simulink library "carnot"  (R2018b)
settings: Solver=VariableStepAuto  StartTime=0.0  StopTime=10.0  RelTol=1e-3
undefined symbols (not defined in the file or in its folder): A, A_earth, acol, Acol, ActPower1, ActPower2, ActPower3, Ad, Ad0, Ar, Au, Au0, Azimuth_Angle, B, Bd, Bd0, Br, Bu, Bu0, C, c1, c2, c3, c33, c4, c5, c6, CarnotCallbacks_Density, CarnotCallbacks_Enthalpy, CarnotCallbacks_Enthalpy2Temperature, CarnotCallbacks_Entropy, CarnotCallbacks_Evaporation_Enthalpy, CarnotCallbacks_GlobalMessageLevel, CarnotCallbacks_Grashof, CarnotCallbacks_Heat_Capacity, CarnotCallbacks_Kinematic_Viscosity, CarnotCallbacks_PMV_PPD, CarnotCallbacks_Prandtl, CarnotCallbacks_Saturation_Property, CarnotCallbacks_Saturation_Temperature, CarnotCallbacks_Saturation_Value_Water, CarnotCallbacks_Specific_Volume, CarnotCallbacks_Thermal_Conductivity, CarnotCallbacks_Vapour_Content, CarnotCallbacks_Vapour_Pressure, Cd, Cdl, Cr, Cu, Davies, Dd, DE_TRY2010_04_averageYear, delta_grd, density, DiameterLastPiece, dl, DPConstant, DPLinear, DPQuadratic, Dr ... (+59)
libraries: $bdroot x429, simulink x36, simulink_extras x12
(part 20 of 22)

== system carnot/Source/Chiller/Absorption_Chiller_ddT/boiler ==
  THBhot_in : Inport
  deltadelta_t : Inport  Port=2
  on : Inport  Port=3
  Bus Assignment : BusAssignment  AssignedSignals=Temperature
  Bus Selector : BusSelector  OutputSignals=Temperature,MassFlow,Pressure,FluidType,FluidMix
  Pressure_Drop_Fix : $bdroot/Basic/Pressure_Drop/Pressure_Drop_Fix  con=0  lin=dpg(1)  qua=dpg(2)
  Qdot_G with deltadelta_t : Subsystem
  Thot_out : Subsystem
  prod : Product
  THVhot_out : Outport
  t_B : Outport  Port=2
  Qdot_G [W] : Outport  Port=3
  wires:
  Pressure_Drop_Fix/1 -> THVhot_out/1
  Thot_out/1(Thot_out) -> Bus Assignment/2
  Bus Assignment/1 -> Pressure_Drop_Fix/1
  THBhot_in/1 -> Bus Assignment/1, Bus Selector/1
  Qdot_G with deltadelta_t/1(Qdot_G [W]) -> prod/2
  on/1 -> prod/1
  prod/1 -> Qdot_G [W]/1, Thot_out/3(Qdot_G)
  deltadelta_t/1 -> Qdot_G with deltadelta_t/1(deltadelta_t)
  Bus Selector/5 -> Thot_out/6(mix)  "<FluidMix>"
  Bus Selector/4 -> Thot_out/5(fluid)  "<FluidType>"
  Bus Selector/3 -> Thot_out/4(p)  "<Pressure>"
  Bus Selector/1 -> t_B/1, Thot_out/1(Thot_in)  "<Temperature>"
  Bus Selector/2 -> Thot_out/2(mdot)  "<MassFlow>"

== system carnot/Source/Chiller/Absorption_Chiller_ddT/deltadelta_t ==
  note: deltadelta_t = t_B - (1+E) * t_AC + E * t_E
  t_B : Inport
  t_E : Inport  Port=2
  t_AC : Inport  Port=3
  Add : Sum  Inputs=++-
  Gain : Gain  Gain=1+E
  Gain1 : Gain  Gain=E
  deltadelta_t : Outport
  wires:
  t_AC/1 -> Gain/1
  t_E/1 -> Gain1/1
  Add/1 -> deltadelta_t/1
  t_B/1 -> Add/1
  Gain1/1 -> Add/2
  Gain/1 -> Add/3

== system carnot/Source/Chiller/Absorption_Chiller_ddT/evaporator ==
  THBload_in : Inport
  deltadelta_t : Inport  Port=2
  on : Inport  Port=3
  Bus Assignment : BusAssignment  AssignedSignals=Temperature
  Bus Selector : BusSelector  OutputSignals=Temperature,MassFlow,Pressure,FluidType,FluidMix
  Pressure_Drop_Fix : $bdroot/Basic/Pressure_Drop/Pressure_Drop_Fix  con=0  lin=dpe(1)  qua=dpe(2)
  Qdot_E with deltadelta_t : Subsystem
  Tchilled_out : Subsystem
  prod : Product
  THBload : Outport
  t_E : Outport  Port=2
  Qdot_E [W] : Outport  Port=3
  wires:
  Pressure_Drop_Fix/1 -> THBload/1
  Bus Assignment/1 -> Pressure_Drop_Fix/1
  THBload_in/1 -> Bus Assignment/1, Bus Selector/1
  Qdot_E with deltadelta_t/1(Qdot_E [W]) -> prod/2
  prod/1 -> Qdot_E [W]/1, Tchilled_out/3(Qdot_E)
  on/1 -> prod/1
  Bus Selector/3 -> Tchilled_out/4(p)  "<Pressure>"
  Tchilled_out/1(Tcold) -> Bus Assignment/2, t_E/1
  deltadelta_t/1 -> Qdot_E with deltadelta_t/1(deltadelta_t)
  Bus Selector/5 -> Tchilled_out/6(mix)  "<FluidMix>"
  Bus Selector/4 -> Tchilled_out/5(fluid)  "<FluidType>"
  Bus Selector/1 -> Tchilled_out/1(T)  "<Temperature>"
  Bus Selector/2 -> Tchilled_out/2(mdot)  "<MassFlow>"

== system carnot/Source/Chiller/Compression_Air_Water_Chiller/Lookup_tables _COP + Q_cold_faktor ==
  T_AIR_IN : Inport
  T_WATER_OUT : Inport  Port=2
  control_AC : Inport  Port=3
  Constant : Constant  Value=Q_Nom
  Gain : Gain  Gain=1000
  Product : Product  RndMeth=Zero
  Product1 : Product  Inputs=4  RndMeth=Zero
  Product2 : Product  Inputs=/*  RndMeth=Zero
  lookup_table_COP : Lookup_n-D  BreakpointsForDimension1=[7,18]  BreakpointsForDimension2=[15,20,25,30,35,40]  BreakpointsForDimension3=[1:2]  BreakpointsForDimension4=[1:2]  Table=[3.55 3.15 2.65 2.25 2 1.7;3.8 3.4 2.93 2.58 2.2 1.95]  InputSameDT=on
  lookup_table_Q_cold_faktor : Lookup_n-D  BreakpointsForDimension1=[7,18]  BreakpointsForDimension2=[15,20,25,30,35,40]  BreakpointsForDimension3=[1:2]  BreakpointsForDimension4=[1:2]  Table=|  InputSameDT=on
      | [ 1.26 1.19 1.08 1.00 0.90 0.79;
      |              1.65 1.53 1.41 1.28 1.18 1.09]
  runtime_AC : Subsystem  TreatAsAtomicUnit=on
      mask help: This block counts the time if input is set to one, it stops counting if input is zero and continues when input rises to one again.
      mask Help: eval('filetest (''manual.htm#count_working_time'')')
  start-up-faktor : Fcn  Expr=1-exp(-u/(150/5))
  COP : Outport
  Q_cold : Outport  Port=2
  P_el : Outport  Port=3
  wires:
  Gain/1 -> Q_cold/1, Product2/2
  T_WATER_OUT/1 -> lookup_table_Q_cold_faktor/1, lookup_table_COP/1
  T_AIR_IN/1 -> lookup_table_Q_cold_faktor/2, lookup_table_COP/2
  lookup_table_COP/1 -> Product/1, Product2/1
  control_AC/1 -> Product/2, runtime_AC/1(control_AC), Product1/2
  lookup_table_Q_cold_faktor/1 -> Product1/3
  runtime_AC/1(runtime) -> start-up-faktor/1
  Product/1 -> COP/1
  Product1/1 -> Gain/1
  start-up-faktor/1 -> Product1/1
  Constant/1 -> Product1/4
  Product2/1 -> P_el/1

== system carnot/Source/Chiller/Compression_Air_Water_Chiller/cooling ==
  THB_in : Inport
  Q_cold : Inport  Port=2
  Bus Assignment : BusAssignment  AssignedSignals=Temperature
  Bus Selector : BusSelector  OutputSignals=Temperature,MassFlow
  Constant : Constant  Value=20
  Constant_THB : $bdroot/Source/Simple/Constant_THB  t=40  mdot=0*100/3600  p=1e5  mID=No Pressure Drop  fluid=Water  mix=0  mix2=0  mix3=0  dia=0.02  hgt=0
  Ground : Ground
  Heat_Capacity : $bdroot/Basic/Material_Properties/Heat_Capacity  VariantControl=CarlibClassic  INPUTARGUMENTS=THB  DEBUGLEVEL=DEBUGLEVEL  MAXTOTALWARNINGS=inf  MAXCONSECUTIVEWARNINGS=inf  WRITETOFILE=0  FILENAME='errors.txt'
  Product : Product  Inputs=//*  SaturateOnIntegerOverflow=on  RndMeth=Zero  InputSameDT=on  OutDataTypeStr=Inherit: Same as first input
  Saturation : Saturate  UpperLimit=inf  LowerLimit=1
  Storage_Type_1 : $bdroot/Storage/Thermal/Storage_Type_1  t0=20  hgt=1.7684  stgtype=1  tini=[20 20 20 20 20 20 20 20 20 20]  mpts=[1 2 3 4 5 6 7 8 9 10]  PathName=fullfile(path_carnot('libsl'), 'Storage', 'Thermal', 'Storage_Type_1', 'parameter_set')  FileName='StorageType1_500_L.mat'  userPath=off  userParam=off  uwall=1  ubot=1  utop=1  axcond=1  volume=0.5  dia=0.6  standing=standing cylinder  nodes=10  mpoints=10  Tsensor=0.5  pipe1inlet=1  pipe1outlet=0  pipe1dia=0.03  pipe2inlet=0  pipe2outlet=1  pipe2dia=0.03  heater1start=0.6  heater1end=0.65
  Sum2 : Sum  Inputs=+-  InputSameDT=on  OutDataTypeStr=Inherit: Same as first input
  Terminator : Terminator
  Terminator1 : Terminator
  Terminator2 : Terminator
  isinf : MATLAB Function  TreatAsAtomicUnit=on
  isnan : MATLAB Function  TreatAsAtomicUnit=on
  THB_out : Outport
  wires:
  Ground/1 -> Storage_Type_1/4
  Storage_Type_1/3 -> Terminator2/1
  Storage_Type_1/2 -> Terminator1/1
  Storage_Type_1/1 -> Terminator/1
  Storage_Type_1/4 -> THB_out/1
  Bus Selector/2 -> Product/1  "<MassFlow>"
  Heat_Capacity/1 -> Product/2
  Bus Assignment/1 -> Storage_Type_1/3
  Constant/1 -> Storage_Type_1/1
  Constant_THB/1 -> Storage_Type_1/2
  THB_in/1 -> Heat_Capacity/1, Bus Selector/1, Bus Assignment/1
  Bus Selector/1 -> Sum2/1  "<Temperature>"
  Q_cold/1 -> Product/3  "W"
  isnan/1(y) -> isinf/1(u)
  Product/1 -> isnan/1(u)
  isinf/1(y) -> Sum2/2
  Sum2/1 -> Saturation/1
  Saturation/1 -> Bus Assignment/2

== system carnot/Source/Chiller/Compression_Air_Water_Chiller/measure_T_WATER_OUT ==
  THV_in : Inport
  Demux3 : Demux  Outputs=2
  Terminator : Terminator
  heat capacity : StateSpace  A=-tc  B=tc  D=0  InitialCondition=t0
  select temperature : Selector  InputPortWidth=5  IndexOptions=Index vector (dialog)  Indices=[2]  OutputSizes=1
  T : Outport
  THV : Outport  Port=2
  wires:
  Demux3/2 -> Terminator/1
  Demux3/1 -> select temperature/1
  THV_in/1 -> Demux3/1, THV/1
  select temperature/1 -> heat capacity/1
  heat capacity/1 -> T/1

== system carnot/Source/Chiller/Cooling_Tower/Fan ==
  note: Grundlage zur Berechnung
      | bei Drehzahländerung eines bestimmten Lüfters
      |
      | Proportionalitätsgesetz
      | V1/V2 = n1/n2
      | P1/P2 = (n1/n2)^3
      |
      | Wirkungsgrad Elektromotor
      | P = Pm/eta
  n_fan : Inport
  Divide1 : Product  Inputs=*/
  Divide2 : Product  Inputs=*/*
  Divide3 : Product  Inputs=/*
  Divide4 : Product  Inputs=/*
  Input Leistung : Constant  Value=1.8
  Math Function : Math  Operator=pow  SaturateOnIntegerOverflow=on
  Pw1 : Constant  Value=3
  max. Drehzahl : Constant  Value=824
  max. Vdot_Lüfter : Constant  Value=2.2
  n_fan [%] : Outport
  vdot_fan : Outport  Port=2
  P_fan : Outport  Port=3
  wires:
  n_fan/1 -> Divide2/1, Divide4/1, Divide1/1
  max. Drehzahl/1 -> Divide2/2, Divide1/2, Divide4/2
  Divide1/1 -> n_fan [%]/1
  Input Leistung/1 -> Divide3/2
  max. Vdot_Lüfter/1 -> Divide2/3
  Divide2/1 -> vdot_fan/1
  Divide3/1 -> P_fan/1
  Divide4/1 -> Math Function/1
  Math Function/1 -> Divide3/1
  Pw1/1 -> Math Function/2

== system carnot/Source/Chiller/Cooling_Tower/Feuchtkugel- temperatureinfluss // wet-bulb temperature effect ==
  WDB : Inport
  t_ie : Inport  Port=2
  Enable : EnablePort
  "Abgleich " : Subsystem
  Add : Sum
  Constant : Constant  Value=2
  Divide : Product  Inputs=*/
  THB_WetBulbTemperature : $bdroot/Basic/Material_Properties/THB_WetBulbTemperature
  Terminator1 : Terminator
  WDB2THB : $bdroot/Weather/WDB2THB  dia=0.2
  wet-bulb 15 °C : Subsystem
  t_FK : Outport  InitialOutput=0
  t_ia_FK : Outport  Port=2  InitialOutput=0
  dt : Outport  Port=3  InitialOutput=0
  wires:
  WDB2THB/1 -> THB_WetBulbTemperature/1
  THB_WetBulbTemperature/2 -> Terminator1/1
  WDB/1 -> WDB2THB/1
  wet-bulb 15 °C/1(t_ia_FK15) -> "Abgleich "/3(t_ia_FK15)
  THB_WetBulbTemperature/1 -> "Abgleich "/1(t_FK), t_FK/1
  t_ie/1 -> Add/2, wet-bulb 15 °C/1(t_ie), "Abgleich "/2(t_ie)
  "Abgleich "/1(t_ia_FK) -> Add/1, t_ia_FK/1
  Add/1 -> Divide/1
  Constant/1 -> Divide/2
  Divide/1 -> dt/1

== system carnot/Source/Chiller/Cooling_Tower/Leistungseinflüsse // influence on coolingpower ==
  t_ia_FK : Inport
  cp_i : Inport  Port=2
  t_ie : Inport  Port=3
  mdot_i : Inport  Port=4
  Fluid_Type : Inport  Port=5
  Fluid_mix : Inport  Port=6
  n_fan [%] : Inport  Port=7
  Enable : EnablePort
  Qdot_i_FK : Subsystem
  "Qdot_i_ist " : Subsystem
  "t_ia_ist " : Subsystem
  Qdot_i_ist : Outport  InitialOutput=0
  t_ia_ist : Outport  Port=2  InitialOutput=0
  wires:
  "Qdot_i_ist "/1(Qdot_i_ist) -> Qdot_i_ist/1, "t_ia_ist "/1(Qdot_i_ist)
  Qdot_i_FK/1(Qdot_i_FK) -> "Qdot_i_ist "/1(Qdot_i_FK)
  t_ie/1 -> Qdot_i_FK/2(t_ie), "t_ia_ist "/2(t_ie), "Qdot_i_ist "/6(t_ie)
  t_ia_FK/1 -> Qdot_i_FK/1(t_ia_FK)
  n_fan [%]/1 -> "Qdot_i_ist "/2(n_Fan [%])
  "t_ia_ist "/1(t_ia_ist) -> t_ia_ist/1
  cp_i/1 -> "t_ia_ist "/3(cp_i)
  Fluid_Type/1 -> Qdot_i_FK/3(Fluid_Type), "Qdot_i_ist "/5(Fluid_Type)
  mdot_i/1 -> "Qdot_i_ist "/4(mdot_i), "t_ia_ist "/4(mdot)
  Fluid_mix/1 -> "Qdot_i_ist "/3(Fluid_mix)

== system carnot/Source/Chiller/Cooling_Tower/Verbrauch // consumption ==
  Qdot : Inport
  vdot_fan : Inport  Port=2
  P_fan : Inport  Port=3
  control_fan : Inport  Port=4
  phi_le : Inport  Port=5
  t_le : Inport  Port=6
  t_ie : Inport  Port=7
  Strom : Subsystem
  Verdunstung : Subsystem
  energy : Outport
  power : Outport  Port=2
  Wasserverbrauch : Outport  Port=3
  wires:
  control_fan/1 -> Strom/1(control_Fan), Verdunstung/1(control_Fan)
  P_fan/1 -> Strom/2(P_Fan)
  Strom/2(power) -> power/1
  t_le/1 -> Verdunstung/2(t_le)
  Verdunstung/1(Wasserverbrauch) -> Wasserverbrauch/1
  phi_le/1 -> Verdunstung/3(phi_le)
  vdot_fan/1 -> Verdunstung/4(Vdot_Fan)
  Qdot/1 -> Verdunstung/5(Qdot)
  t_ie/1 -> Verdunstung/6(t_ie)
  Strom/1(energy) -> energy/1

== system carnot/Source/Cogeneration/microCHP_constant/energy and efficiency ==
  P_th : Inport
  control_CHP : Inport  Port=2
  P_gas : Inport  Port=3
  P_el : Inport  Port=4
  Add : Sum
  Dot Product1 : DotProduct  InputSameDT=on  OutDataTypeStr=Inherit: Inherit via internal rule
  Dot Product2 : DotProduct  InputSameDT=on  OutDataTypeStr=Inherit: Inherit via internal rule
  Dot Product4 : DotProduct  InputSameDT=on  OutDataTypeStr=Inherit: Inherit via internal rule
  Integrator : Integrator
  Integrator1 : Integrator
  Integrator2 : Integrator
  Product1 : Product  Inputs=*/  SaturateOnIntegerOverflow=on  RndMeth=Zero  InputSameDT=on  OutDataTypeStr=Inherit: Same as first input
  Product2 : Product  Inputs=/*  SaturateOnIntegerOverflow=on  RndMeth=Zero  InputSameDT=on  OutDataTypeStr=Inherit: Same as first input
  Q_th : Outport
  Q_el : Outport  Port=2
  Q_Gas : Outport  Port=3
  eta_th : Outport  Port=4
  eta_el : Outport  Port=5
  eta_sys : Outport  Port=6
  wires:
  Add/1 -> eta_sys/1
  Product1/1 -> eta_th/1, Add/1
  Integrator1/1 -> Q_th/1, Product1/1
  P_th/1 -> Dot Product1/1
  Dot Product1/1 -> Integrator1/1
  Integrator2/1 -> Q_el/1, Product2/2
  Integrator/1 -> Product1/2, Q_Gas/1, Product2/1
  control_CHP/1 -> Dot Product1/2, Dot Product4/1, Dot Product2/1
  Dot Product2/1 -> Integrator/1
  Dot Product4/1 -> Integrator2/1
  Product2/1 -> Add/2, eta_el/1
  P_el/1 -> Dot Product4/2
  P_gas/1 -> Dot Product2/2

== system carnot/Source/Cogeneration/microCHP_constant/measure_T ==
  THV_in : Inport
  heat capacity : StateSpace  A=-tc  B=tc  D=0  InitialCondition=t0
  select temperature : Selector  InputPortWidth=20  IndexOptions=Index vector (dialog)  Indices=[2]  OutputSizes=1
  THV : Outport
  T : Outport  Port=2
  wires:
  heat capacity/1 -> T/1
  select temperature/1 -> heat capacity/1
  THV_in/1 -> THV/1, select temperature/1

== system carnot/Source/Cogeneration/microCHP_constant/pump and return temperature raising facility ==
  note: heating power
  THVin : Inport
  control : Inport  Port=2
  " " : Constant  Value=P_th
  " ." : Product  Inputs=*/
  " .  " : Sum  Inputs=-+
  . : Sum  Inputs=-+
  ". " : Product  Inputs=*/
  Demux : Demux  Outputs=[1 1 18]
  Divide1 : Product  Inputs=****
  Ground : Ground
  Mux1 : Mux  Inputs=[1 1 1 7 10]
  P_th_base : Constant  Value=11520
  T_flow-lookup table : Lookup_n-D  NumberOfTableDimensions=1  BreakpointsForDimension1=[45,50,60,65,74]  BreakpointsForDimension2=[44,80]  BreakpointsForDimension3=[1:2]  BreakpointsForDimension4=[1:2]  Table=[78.5 79.65 81 84.18 92.47]  InputSameDT=on
  T_flow_setpoint : Constant  Value=T_flow_setpoint
  const1 : Constant  Value=[p0 fluid_id mix dia 0 0 0]
  heat capacity : Subsystem  mask{NTU=3.3}
      mask prompts: NTU "NTU (k*A/(m*cp))"
  mass flow-lookup table : Lookup_n-D  NumberOfTableDimensions=1  BreakpointsForDimension1=[45,50,60,65,74]  BreakpointsForDimension2=[44,80]  BreakpointsForDimension3=[1:2]  BreakpointsForDimension4=[1:2]  Table=[0.09 0.1 0.129 0.139 0.140]  InputSameDT=on
  terminate1 : Terminator
  THV : Outport
  wires:
  control/1 -> Divide1/4
  " ."/1 -> Divide1/3  "f_power"
  ". "/1 -> Divide1/2  "f_flowSetpoint"
  P_th_base/1 -> " ."/2
  T_flow-lookup table/1 -> ./2
  T_flow_setpoint/1 -> " .  "/2
  " .  "/1 -> ". "/2
  ./1 -> ". "/1
  Divide1/1 -> Mux1/3  "mdot"
  mass flow-lookup table/1 -> Divide1/1
  " "/1 -> " ."/1
  THVin/1 -> Demux/1
  const1/1 -> Mux1/4
  Demux/3 -> terminate1/1
  heat capacity/1(T) -> Mux1/2
  Demux/2 -> " .  "/1, T_flow-lookup table/1, ./1, mass flow-lookup table/1, heat capacity/1(Tin)  "T"
  Mux1/1 -> THV/1
  Demux/1 -> Mux1/1  "ID"
  Ground/1 -> Mux1/5  "not used"

== system carnot/Source/Cogeneration/microCHP_modulating/Control_Unit ==
  note: T_flow_ctrl
  cp : Inport
  mdot_return : Inport  Port=2
  T_flow : Inport  Port=3
  demand_control : Inport  Port=4
  T_return_load : Inport  Port=5
  Add : Sum  Inputs=+-
  Constant1 : Constant  Value=60
  Constant10 : Constant  Value=T_flow_setpoint
  Constant6 : Constant
  Constant7 : Constant  Value=t_start
  Constant8 : Constant  Value=P_th_start
  Constant9 : Constant  Value=P_th_max
  Integrator : Integrator  ExternalReset=level
  Logical Operator1 : Logic  Operator=NOT  AllPortsSameDT=off  OutDataTypeStr=boolean
  MinMax : MinMax  Inputs=2
  Product : Product
  Product1 : Product  Inputs=3
  Relational Operator : RelationalOperator  Operator=>  OutDataTypeStr=boolean  RndMeth=Simplest
  Relational Operator1 : RelationalOperator  Operator=>  OutDataTypeStr=boolean  RndMeth=Simplest
  Relay : Relay  OnSwitchValue=T_flow_max  OffSwitchValue=T_flow_max-1  OnOutputValue=0  OffOutputValue=1
  Saturation : Saturate  UpperLimit=P_th_max  LowerLimit=P_th_min
  Switch1 : Switch  Criteria=u2 ~= 0
  Switch2 : Switch  Criteria=u2 ~= 0
  control_CHP : Outport
  P_th : Outport  Port=2
  wires:
  T_return_load/1 -> Add/2
  cp/1 -> Product1/2
  Product/1 -> P_th/1
  mdot_return/1 -> Product1/1
  demand_control/1 -> MinMax/2
  T_flow/1 -> Relay/1, Relational Operator/1
  Add/1 -> Product1/3
  Relay/1 -> MinMax/1
  MinMax/1 -> control_CHP/1, Product/2, Logical Operator1/1
  Constant1/1 -> Relational Operator/2
  Relational Operator/1 -> Switch1/2
  Saturation/1 -> Switch1/1  "Pth_setpoint"
  Constant6/1 -> Integrator/1
  Logical Operator1/1 -> Integrator/2
  Integrator/1 -> Relational Operator1/1
  Constant7/1 -> Relational Operator1/2
  Relational Operator1/1 -> Switch2/2
  Constant8/1 -> Switch2/3
  Constant9/1 -> Switch1/3
  Switch1/1 -> Switch2/1
  Constant10/1 -> Add/1
  Product1/1 -> Saturation/1
  Switch2/1 -> Product/1

== system carnot/Source/Cogeneration/microCHP_modulating/energy and efficiency ==
  control CHP : Inport
  P_th : Inport  Port=2
  P_gas : Inport  Port=3
  P_el : Inport  Port=4
  Add : Sum
  Dot Product1 : DotProduct  InputSameDT=on  OutDataTypeStr=Inherit: Inherit via internal rule
  Dot Product2 : DotProduct  InputSameDT=on  OutDataTypeStr=Inherit: Inherit via internal rule
  Dot Product4 : DotProduct  InputSameDT=on  OutDataTypeStr=Inherit: Inherit via internal rule
  Integrator : Integrator
  Integrator1 : Integrator
  Integrator2 : Integrator
  Product1 : Product  Inputs=*/  SaturateOnIntegerOverflow=on  RndMeth=Zero  InputSameDT=on  OutDataTypeStr=Inherit: Same as first input
  Product2 : Product  Inputs=/*  SaturateOnIntegerOverflow=on  RndMeth=Zero  InputSameDT=on  OutDataTypeStr=Inherit: Same as first input
  Q_th : Outport
  Q_el : Outport  Port=2
  Q_gas : Outport  Port=3
  eta_th : Outport  Port=4
  eta_el : Outport  Port=5
  eta_sys : Outport  Port=6
  wires:
  P_gas/1 -> Dot Product2/2
  P_el/1 -> Dot Product4/2
  Product2/1 -> eta_el/1, Add/2
  Dot Product4/1 -> Integrator2/1
  Dot Product2/1 -> Integrator/1
  control CHP/1 -> Dot Product2/1, Dot Product4/1, Dot Product1/2
  Integrator/1 -> Product2/1, Q_gas/1, Product1/2
  Integrator2/1 -> Product2/2, Q_el/1
  Dot Product1/1 -> Integrator1/1
  P_th/1 -> Dot Product1/1
  Integrator1/1 -> Product1/1, Q_th/1
  Product1/1 -> Add/1, eta_th/1
  Add/1 -> eta_sys/1

== system carnot/Source/Cogeneration/microCHP_modulating/measure_T ==
  THV_in : Inport
  heat capacity : StateSpace  A=-tc  B=tc  D=0  InitialCondition=t0
  select temperature : Selector  InputPortWidth=20  IndexOptions=Index vector (dialog)  Indices=[2]  OutputSizes=1
  T : Outport
  THV : Outport  Port=2
  wires:
  THV_in/1 -> select temperature/1, THV/1
  select temperature/1 -> heat capacity/1
  heat capacity/1 -> T/1

== system carnot/Source/Cogeneration/microCHP_modulating/measure_mdot ==
  THV_in : Inport
  select massflow : Selector  InputPortWidth=20  IndexOptions=Index vector (dialog)  Indices=[3]  OutputSizes=1
  THV : Outport
  mdot : Outport  Port=2
  wires:
  THV_in/1 -> select massflow/1, THV/1
  select massflow/1 -> mdot/1

== system carnot/Source/Cogeneration/microCHP_modulating/pump_const ==
  note: maximum power
  note: nominal power of basic unit
  THVin : Inport
  control : Inport  Port=2
  Constant : Constant  Value=P_th_max
  Constant2 : Constant  Value=12500
  Demux1 : Demux  Outputs=[1 1 18]
  Ground : Ground
  ID : Constant
  Mux1 : Mux  Inputs=[1 1 1 7 10]
  Product1 : Product  Inputs=**/  SaturateOnIntegerOverflow=on  RndMeth=Zero  InputSameDT=on  OutDataTypeStr=Inherit: Same as first input
  Terminator : Terminator
  const1 : Constant  Value=[p0 fluid_id mix dia 0 0 0]
  heat capacity : Subsystem  mask{NTU=3.1}
      mask prompts: NTU "NTU (k*A/(m*cp))"
  mdot : Gain  Gain=mdotmax  SaturateOnIntegerOverflow=on  OutDataTypeStr=Inherit: Same as input  ParamDataTypeStr=Inherit: Same as input
  terminate : Terminator
  THV : Outport
  wires:
  Ground/1 -> Mux1/5  "not used"
  Demux1/3 -> terminate/1
  THVin/1 -> Demux1/1
  ID/1 -> Mux1/1  "ID"
  Mux1/1 -> THV/1
  const1/1 -> Mux1/4
  Demux1/1 -> Terminator/1  "ID"
  Demux1/2 -> heat capacity/1(Tin)  "T"
  mdot/1 -> Product1/2
  Constant/1 -> Product1/1
  Constant2/1 -> Product1/3
  Product1/1 -> Mux1/3
  heat capacity/1(T) -> Mux1/2  "T"
  control/1 -> mdot/1

== system carnot/Source/Cogeneration/microCHP_modulating/return temperature raising facility ==
  THB_flow : Inport
  P_th : Inport  Port=2
  THB_return_load : Inport  Port=3
  . : Product  Inputs=//*  SaturateOnIntegerOverflow=on  RndMeth=Zero  InputSameDT=on  OutDataTypeStr=Inherit: Same as first input
  Add : Sum  Inputs=+-
  Bus Selector : BusSelector  OutputSignals=MassFlow,Temperature,Pressure,FluidType,FluidMix
  Constant1 : Constant  Value=T_flow_setpoint
  Constant3 : Constant  Value=0
  Flow_Diverter : $bdroot/Hydraulics/Flow_Diverter
  Flow_Mixer_Thermostatic : $bdroot/Hydraulics/Flow_Mixer_Thermostatic  t=1
  Heat_Capacity : $bdroot/Basic/Material_Properties/Heat_Capacity  VariantControl=CarlibClassic  INPUTARGUMENTS=state variables (classic)  DEBUGLEVEL=DEBUGLEVEL  MAXTOTALWARNINGS=inf  MAXCONSECUTIVEWARNINGS=inf  WRITETOFILE=0  FILENAME='errors.txt'
  Switch : Switch  Threshold=1  SaturateOnIntegerOverflow=on  InputSameDT=on
  THB_return : Outport
  THB_flow_load : Outport  Port=2
  wires:
  P_th/1 -> ./3, Switch/2
  Heat_Capacity/1 -> ./2
  Bus Selector/2 -> Heat_Capacity/1  "<Temperature>"
  Bus Selector/1 -> ./1  "<MassFlow>"
  Bus Selector/5 -> Heat_Capacity/4  "<FluidMix>"
  Bus Selector/4 -> Heat_Capacity/3  "<FluidType>"
  Bus Selector/3 -> Heat_Capacity/2  "<Pressure>"
  Flow_Diverter/2 -> THB_flow_load/1
  THB_return_load/1 -> Flow_Mixer_Thermostatic/2
  Constant1/1 -> Add/1
  Add/1 -> Switch/1
  ./1 -> Add/2
  Constant3/1 -> Switch/3
  Switch/1 -> Flow_Mixer_Thermostatic/4
  THB_flow/1 -> Flow_Diverter/1, Bus Selector/1
  Flow_Mixer_Thermostatic/2 -> Flow_Diverter/2
  Flow_Mixer_Thermostatic/1 -> THB_return/1
  Flow_Diverter/1 -> Flow_Mixer_Thermostatic/1
  Flow_Diverter/3 -> Flow_Mixer_Thermostatic/3

== system carnot/Source/Cogeneration/microCHP_modulating/scale_function ==
  P_th : Inport
  . : Sum  Inputs=+-
  .1 : Sum  Inputs=-+
  Add : Sum
  Divide : Product  Inputs=*/
  b : Constant  Value=P_th_max
  m : Constant  Value=P_th_min
  m2 : Constant
  X_pth : Outport
  wires:
  m2/1 -> Add/2
  m/1 -> ./2, .1/1
  ./1 -> Divide/1
  b/1 -> .1/2
  .1/1 -> Divide/2
  P_th/1 -> ./1
  Divide/1 -> Add/1
  Add/1 -> X_pth/1

== system carnot/Source/Heat_Exchanger/Radiator_AIV/Troom ==
  "[AIV]" : Inport
  Sum4 : Sum  Inputs=1  SaturateOnIntegerOverflow=on  InputSameDT=on  OutDataTypeStr=Inherit: Same as first input
  gain : Gain  Gain=0.5  SaturateOnIntegerOverflow=on  OutDataTypeStr=Inherit: Same as input  ParamDataTypeStr=Inherit: Same as input
  select Tc Tr : Selector  InputPortWidth=9  IndexOptions=Index vector (dialog)  Indices=[2 3]  OutputSizes=1
  Troom : Outport
  wires:
  select Tc Tr/1 -> Sum4/1
  Sum4/1 -> gain/1
  gain/1 -> Troom/1  "Troom"
  "[AIV]"/1 -> select Tc Tr/1

== system carnot/Source/Heat_Pump/Ground_Source_Heat_Exchanger/BoundaryCondition1 ==
  note: virtual fluid temperature node T_Earth(i,0) is the
      | fluid temperature that would pull the thermal
      | power through the resistance L1 (= average of
      | Tup and Tdown)
  T_Up : Inport
  T_Down : Inport  Port=2
  T_Earth(i,1) : Inport  Port=3
  Gain : Gain  Gain=1/dl
  Gain1 : Gain  Gain=L1/2  SaturateOnIntegerOverflow=on  OutDataTypeStr=Inherit: Same as input  ParamDataTypeStr=Inherit: Same as input
  Gain2 : Gain  Gain=L1/2  SaturateOnIntegerOverflow=on  OutDataTypeStr=Inherit: Same as input  ParamDataTypeStr=Inherit: Same as input
  Gain3 : Gain  Gain=1/L1  SaturateOnIntegerOverflow=on  OutDataTypeStr=Inherit: Same as input  ParamDataTypeStr=Inherit: Same as input
  Sum3 : Sum  Inputs=|-+  SaturateOnIntegerOverflow=on  InputSameDT=on  OutDataTypeStr=Inherit: Same as first input
  Sum4 : Sum  Inputs=|-+  SaturateOnIntegerOverflow=on  InputSameDT=on  OutDataTypeStr=Inherit: Same as first input
  Sum5 : Sum  Inputs=|++  SaturateOnIntegerOverflow=on  InputSameDT=on  OutDataTypeStr=Inherit: Same as first input
  Sum6 : Sum  Inputs=|-+  SaturateOnIntegerOverflow=on  InputSameDT=on  OutDataTypeStr=Inherit: Same as first input
  T_Earth(i,0) : Outport
  qdot,i : Outport  Port=2
  wires:
  Gain/1 -> qdot,i/1
  Sum6/1 -> T_Earth(i,0)/1
  T_Earth(i,1)/1 -> Sum4/2, Sum6/2, Sum3/2
  T_Up/1 -> Sum4/1
  T_Down/1 -> Sum3/1
  Gain3/1 -> Sum6/1  "dT"
  Sum5/1 -> Gain3/1, Gain/1  "Qtot,i"
  Gain2/1 -> Sum5/2  "Qup,i"
  Gain1/1 -> Sum5/1  "Qdown,i"
  Sum4/1 -> Gain2/1
  Sum3/1 -> Gain1/1

== system carnot/Source/Heat_Pump/Ground_Source_Heat_Exchanger/BoundaryCondition2 ==
  note: T_Earth(i,DimRad)
  qdot,i : Inport
  Dd6 : Gain  Gain=c4  Multiplication=Matrix(K*u)  SaturateOnIntegerOverflow=on  OutDataTypeStr=Inherit: Same as input  ParamDataTypeStr=Inherit: Same as input
  Sum2 : Sum  Inputs=|+-  SaturateOnIntegerOverflow=on  InputSameDT=on  OutDataTypeStr=Inherit: Same as first input
  Tearth DimRad : Constant  Value=T_null  VectorParams1D=off
  g-function : Subsystem
  T_Earth(i,DimRad) Gew : Outport
  T_Earth(i,DimRad) : Outport  Port=2
  wires:
  Sum2/1 -> Dd6/1, T_Earth(i,DimRad)/1
  Tearth DimRad/1 -> Sum2/1
  qdot,i/1 -> g-function/1(qdot,i)
  Dd6/1 -> T_Earth(i,DimRad) Gew/1
  g-function/1(DeltaT) -> Sum2/2  "DeltaT"

== system carnot/Source/Heat_Pump/Ground_Source_Heat_Exchanger/Tdown ==
  note: instationary calculation of Tdown (Huber 1997)
  Tin,TEarth : Inport
  A mult : Product  Multiplication=Matrix(*)  RndMeth=Zero
  B mult : Product  Multiplication=Matrix(*)  RndMeth=Zero
  C mult : Product  Multiplication=Matrix(*)  RndMeth=Zero
  D mult : Product  Multiplication=Matrix(*)  RndMeth=Zero
  Integrator : Integrator  InitialCondition=Tdown_0
  Sum1 : Sum  Inputs=|++
  Sum2 : Sum  Inputs=++|
  Tdown : Outport
  wires:
  Sum2/1 -> Tdown/1  "y"
  Tin,TEarth/1 -> B mult/2, D mult/2
  D mult/1 -> Sum2/1
  C mult/1 -> Sum2/2
  B mult/1 -> Sum1/1
  Sum1/1 -> Integrator/1  "Xdot"
  Integrator/1 -> A mult/2, C mult/2  "X"
  A mult/1 -> Sum1/2
  [B] -> B mult/1
  [A] -> A mult/1
  [C] -> C mult/1
  [D] -> D mult/1

== system carnot/Source/Heat_Pump/Ground_Source_Heat_Exchanger/Tup ==
  note: instationary calculation of Tup (Huber 1997)
  Tin,TEarth : Inport
  A mult : Product  Multiplication=Matrix(*)  RndMeth=Zero
  B mult : Product  Multiplication=Matrix(*)  RndMeth=Zero
  C mult : Product  Multiplication=Matrix(*)  RndMeth=Zero
  D mult : Product  Multiplication=Matrix(*)  RndMeth=Zero
  Integrator : Integrator  InitialCondition=Tup_0
  Sum1 : Sum  Inputs=|++
  Sum2 : Sum  Inputs=++|
  Tup : Outport
  wires:
  Sum2/1 -> Tup/1  "y"
  Tin,TEarth/1 -> B mult/2, D mult/2
  D mult/1 -> Sum2/1
  C mult/1 -> Sum2/2
  B mult/1 -> Sum1/1
  Sum1/1 -> Integrator/1  "Xdot"
  Integrator/1 -> A mult/2, C mult/2  "X"
  A mult/1 -> Sum1/2
  [Bu] -> B mult/1
  [Au] -> A mult/1
  [Cu] -> C mult/1
  [Du] -> D mult/1

== system carnot/Source/Solar_Thermal/Collector_1xN/create_Cdat ==
  acol : Inport
  THBin : Inport  Port=2
  THBout : Inport  Port=3
  Qdot : Inport  Port=4
  Tmean : Inport  Port=5
  WDB : Inport  Port=6
  Bus Creator : BusCreator  Inputs=6
  data_c : Outport
  wires:
  Tmean/1 -> Bus Creator/5  "Tmean"
  Qdot/1 -> Bus Creator/4  "Qdot"
  Bus Creator/1 -> data_c/1
  WDB/1 -> Bus Creator/6  "WDB_surface"
  THBout/1 -> Bus Creator/3  "THBout"
  THBin/1 -> Bus Creator/2  "THBin"
  acol/1 -> Bus Creator/1  "Acol"

== system carnot/Source/Solar_Thermal/Collector_Unglazed/Collector_Unglazed ==
  WDB : Inport
  position : Inport  Port=2
  THB_r : Inport  Port=3
  Add : Sum  Inputs=1
  Bus Assignment : BusAssignment  AssignedSignals=Temperature
  Bus Selector : BusSelector  OutputSignals=Solar_Radiation_direct_surface,Solar_Radiation_diffuse_surface,Temperature_Ambient,Temperature_Sky_Radiation,Relative_Humidity,Station_Pressure,Wind_Speed  OutputAsBus=on
  Bus Selector1 : BusSelector  OutputSignals=Temperature,MassFlow,Pressure,FluidType,FluidMix  OutputAsBus=on
  IAM_Table : $bdroot/Source/Solar_Thermal/IncidenceAngleModifier/IAM_Table  fta=fta  angle=[0:5:90]  Kb="[1.0000    1.0000    0.9999    0.9996    0.9991    0.9982    0.9965  0.9935    0.9886    0.9807    0.9678    0.9473    0.9148    0.8638   0.7846    0.6644    0.4907    0.2599    0.0000]"  Kd=0.92
  PowerMeter : $bdroot/Control/PowerMeter
  Pressure_Drop_Collector : $bdroot/Basic/Pressure_Drop/Pressure_Drop_Collector  len=len  lin=lin  qua=qua
  Product : Product  Inputs=*/  RndMeth=Zero
  Radiation_on_Inclined_Surface : $bdroot/Weather/Radiation_on_Inclined_Surface  sky=Perez 1990  reflect=0.2
  Terminator : Terminator
  Width : Width
  const : Constant  Value=acol
  create_Cdat : Subsystem
  unglazed_collector : S-Function  FunctionName=solarcollector_unglazed  Parameters=acol, uc0, uc1, uc0loss, uc1loss, uc0gain, uc1gain, e_sky, uc1eta0, hi, inv_c_abs, inv_c_fl, len, tini, nodes  SFunctionDeploymentMode=off  EnableBusSupport=off
  Cdat : Outport
  THB_s : Outport  Port=2
  wires:
  IAM_Table/1 -> unglazed_collector/2
  Bus Assignment/1 -> Pressure_Drop_Collector/2, PowerMeter/1
  Radiation_on_Inclined_Surface/1 -> create_Cdat/6(WDB), Bus Selector/1, IAM_Table/1
  position/1 -> Pressure_Drop_Collector/3, Radiation_on_Inclined_Surface/2
  WDB/1 -> Radiation_on_Inclined_Surface/1
  THB_r/1 -> Bus Selector1/1, Bus Assignment/1, create_Cdat/2(THBin), PowerMeter/2
  Bus Selector/1 -> unglazed_collector/1
  Bus Selector1/1 -> unglazed_collector/3
  IAM_Table/2 -> Terminator/1
  unglazed_collector/1 -> Bus Assignment/2
  unglazed_collector/2 -> Add/1, Width/1  "Tabsorber"
  const/1 -> create_Cdat/1(acol)
  create_Cdat/1(data_c) -> Cdat/1  "Cdat"
  PowerMeter/1 -> create_Cdat/4(Qdot)
  Add/1 -> Product/1
  Product/1 -> create_Cdat/5(Tmean)
  Width/1 -> Product/2
  Pressure_Drop_Collector/1 -> create_Cdat/3(THBout), THB_s/1  "THB_s"
  unglazed_collector/3 -> Pressure_Drop_Collector/1  "Tfluid"

== system carnot/Source/Solar_Thermal/Collector_Unglazed_ISO9806/create_Cdat ==
  acol : Inport
  THBin : Inport  Port=2
  THBout : Inport  Port=3
  Qdot : Inport  Port=4
  Tmean : Inport  Port=5
  WDB : Inport  Port=6
  Bus Creator : BusCreator  Inputs=6
  data_c : Outport
  wires:
  Tmean/1 -> Bus Creator/5  "Tmean"
  Qdot/1 -> Bus Creator/4  "Qdot"
  Bus Creator/1 -> data_c/1
  WDB/1 -> Bus Creator/6  "WDB_surface"
  THBout/1 -> Bus Creator/3  "THBout"
  THBin/1 -> Bus Creator/2  "THBin"
  acol/1 -> Bus Creator/1  "Acol"

== system carnot/Source/Solar_Thermal/Collector_Unglazed_ISO_2node/Pressure Drop ==
  Tnodes : Inport
  THB : Inport  Port=2
  position : Inport  Port=3
  Bus Assignment : BusAssignment  AssignedSignals=MassFlow
  Bus Assignment1 : BusAssignment  AssignedSignals=MassFlow
  Bus Selector : BusSelector  OutputSignals=MassFlow
  Divide : Product  Inputs=*/
  Ncoll : Constant  Value=Ncollector
  Pressure_Drop_Collector : $bdroot/Basic/Pressure_Drop/Pressure_Drop_Collector  len=len  lin=dplin  qua=dpqua
  THBout : Outport
  wires:
  THB/1 -> Bus Assignment/1, Bus Selector/1
  position/1 -> Pressure_Drop_Collector/3
  Tnodes/1 -> Pressure_Drop_Collector/1
  Pressure_Drop_Collector/1 -> Bus Assignment1/1
  Bus Assignment/1 -> Pressure_Drop_Collector/2
  Bus Selector/1 -> Divide/1, Bus Assignment1/2  "<MassFlow>"
  Divide/1 -> Bus Assignment/2
  Ncoll/1 -> Divide/2
  Bus Assignment1/1 -> THBout/1

== system carnot/Source/Solar_Thermal/Collector_Unglazed_ISO_2node/Tin_node ==
  note: CapAbs/2 * dT/dt = mdot*cp*(Tin-T)
  A*N : Inport
  THB : Inport  Port=2
  Bus Assignment : BusAssignment  AssignedSignals=Temperature
  Bus Selector5 : BusSelector  OutputSignals=Temperature,MassFlow
  Gain : Gain  Gain=2
  Integrator : Integrator  InitialCondition=tini
  Product2 : Product  Inputs=3  RndMeth=Zero
  Product4 : Product  Inputs=*//  RndMeth=Zero
  Subtract3 : Sum  Inputs=-+
  c_abs : Constant  Value=c_abs
  heat_capacity : $bdroot/Basic/Material_Properties/Heat_Capacity  VariantControl=CarlibClassic  INPUTARGUMENTS=THB  DEBUGLEVEL=DEBUGLEVEL  MAXTOTALWARNINGS=inf  MAXCONSECUTIVEWARNINGS=inf  WRITETOFILE=0  FILENAME='errors.txt'
  THB_ : Outport
  wires:
  Product4/1 -> Integrator/1
  THB/1 -> heat_capacity/1, Bus Selector5/1, Bus Assignment/1
  Bus Assignment/1 -> THB_/1
  heat_capacity/1 -> Product2/3
  Bus Selector5/1 -> Subtract3/2  "<Temperature>"
  Bus Selector5/2 -> Product2/2  "<MassFlow>"
  Subtract3/1 -> Product2/1
  Product2/1 -> Gain/1  "power"
  Gain/1 -> Product4/1
  Integrator/1 -> Bus Assignment/2, Subtract3/1  "Tsol"
  c_abs/1 -> Product4/2
  A*N/1 -> Product4/3

== system carnot/Source/Solar_Thermal/Collector_Unglazed_ISO_2node/create_Cdat ==
  acol : Inport
  WDB : Inport  Port=2
  THBin : Inport  Port=3
  THBout : Inport  Port=4
  Qdot : Inport  Port=5
  Tmean : Inport  Port=6
  Bus Creator : BusCreator  Inputs=6
  data_c : Outport
  wires:
  acol/1 -> Bus Creator/1  "Acol"
  THBin/1 -> Bus Creator/2  "THBin"
  THBout/1 -> Bus Creator/3  "THBout"
  WDB/1 -> Bus Creator/6  "WDB_surface"
  Bus Creator/1 -> data_c/1
  Qdot/1 -> Bus Creator/4  "Qdot"
  Tmean/1 -> Bus Creator/5  "Tmean"

== system carnot/Source/Solar_Thermal/IncidenceAngleModifier/IAM_Table ==
  note: q_solar_absorbed = F'(TauAlfa) (Kdir Idir + Kdfu Idfu)
  WDB : Inport
  Bus Selector : BusSelector  OutputSignals=Solar_Radiation_direct_surface,Solar_Radiation_diffuse_surface,Incidence_Angle_sun
  F'(tau*alfa) : Gain  Gain=fta  SaturateOnIntegerOverflow=on  OutDataTypeStr=Inherit: Same as input  ParamDataTypeStr=Inherit: Same as input
  IAM dfu : Gain  Gain=Kd  SaturateOnIntegerOverflow=on  OutDataTypeStr=Inherit: Same as input  ParamDataTypeStr=Inherit: Same as input
  Kb : Lookup  InputValues=angle  Table=Kb  SaturateOnIntegerOverflow=on
  Product1 : Product  SaturateOnIntegerOverflow=on  InputSameDT=on  OutDataTypeStr=Inherit: Same as first input
  Sum1 : Sum  SaturateOnIntegerOverflow=on  InputSameDT=on  OutDataTypeStr=Inherit: Same as first input
  Sum3 : Sum  SaturateOnIntegerOverflow=on  InputSameDT=on  OutDataTypeStr=Inherit: Same as first input
  qsolar : Outport
  Iglb : Outport  Port=2
  wires:
  F'(tau*alfa)/1 -> qsolar/1
  Sum1/1 -> Iglb/1
  Sum3/1 -> F'(tau*alfa)/1
  Kb/1 -> Product1/2
  Bus Selector/3 -> Kb/1  "<Incidence_Angle_sun>"
  Bus Selector/2 -> IAM dfu/1, Sum1/2  "<Solar_Radiation_diffuse_surface>"
  Bus Selector/1 -> Product1/1, Sum1/1  "<Solar_Radiation_direct_surface>"
  IAM dfu/1 -> Sum3/1
  Product1/1 -> Sum3/2
  WDB/1 -> Bus Selector/1

== system carnot/Source/Solar_Thermal/IncidenceAngleModifier/IAM_Table_KbL_KbT ==
  note: q_solar_absorbed = F'(TauAlfa) (Kdir Idir + Kdfu Idfu)
  WDB : Inport
  Abs : Abs
  Abs1 : Abs
  Bus Selector : BusSelector  OutputSignals=Solar_Radiation_direct_surface,Solar_Radiation_diffuse_surface,Incidence_Angle_longitudinal,Incidence_Angle_transversal
  F'(tau*alfa) : Gain  Gain=fta  SaturateOnIntegerOverflow=on  OutDataTypeStr=Inherit: Same as input  ParamDataTypeStr=Inherit: Same as input
  IAM dfu : Gain  Gain=Kd  SaturateOnIntegerOverflow=on  OutDataTypeStr=Inherit: Same as input  ParamDataTypeStr=Inherit: Same as input
  KbL : Lookup  InputValues=kblangle  Table=KbL  SaturateOnIntegerOverflow=on
  KbT : Lookup  InputValues=kbtangle  Table=KbT  SaturateOnIntegerOverflow=on
  Product1 : Product  Inputs=3  SaturateOnIntegerOverflow=on  InputSameDT=on  OutDataTypeStr=Inherit: Same as first input
  Sum1 : Sum  SaturateOnIntegerOverflow=on  InputSameDT=on  OutDataTypeStr=Inherit: Same as first input
  Sum3 : Sum  SaturateOnIntegerOverflow=on  InputSameDT=on  OutDataTypeStr=Inherit: Same as first input
  qsolar : Outport
  Iglb : Outport  Port=2
  wires:
  Abs/1 -> KbT/1
  IAM dfu/1 -> Sum3/1
  F'(tau*alfa)/1 -> qsolar/1
  Sum1/1 -> Iglb/1
  Sum3/1 -> F'(tau*alfa)/1
  KbT/1 -> Product1/3
  KbL/1 -> Product1/2
  Bus Selector/3 -> Abs1/1  "<Incidence_Angle_longitudinal>"
  Bus Selector/4 -> Abs/1  "<Incidence_Angle_transversal>"
  Bus Selector/2 -> IAM dfu/1, Sum1/2  "<Solar_Radiation_diffuse_surface>"
  Bus Selector/1 -> Product1/1, Sum1/1  "<Solar_Radiation_direct_surface>"
  Product1/1 -> Sum3/2
  WDB/1 -> Bus Selector/1
  Abs1/1 -> KbL/1

== system carnot/Source/Solar_Thermal/IncidenceAngleModifier/IAM_b0 ==
  note: teta < 60°: Kdir = 1 - b0 * (1/cos(teta) -1)
      | teta > 60°: Kdir = (1 - b0) * (1 - (teta-60)/30)
  note: q_solar_absorbed = F'(TauAlfa) (Kdir Idir + Kdfu Idfu)
  WDB : Inport
  Bias : Bias  Bias=-1
  Bias1 : Bias  Bias=1
  Bias2 : Bias  Bias=1
  Bias3 : Bias  Bias=-60
  Bias4 : Bias  Bias=1
  Bus Selector : BusSelector  OutputSignals=Incidence_Angle_sun,Solar_Radiation_direct_surface,Solar_Radiation_diffuse_surface
  Compare To Constant : simulink/Logic and Bit Operations/Compare To Constant  relop=>=  const=60  OutDataTypeStr=uint8
  Constant : Constant  Value=1-b0
  Degrees to Radians : simulink_extras/Transformations/Degrees to Radians
  F'(tau*alfa) : Gain  Gain=fta  SaturateOnIntegerOverflow=on  OutDataTypeStr=Inherit: Same as input  ParamDataTypeStr=Inherit: Same as input
  IAM Kdiffuse : Gain  Gain=Kd  SaturateOnIntegerOverflow=on  OutDataTypeStr=Inherit: Same as input  ParamDataTypeStr=Inherit: Same as input
  Math Function : Math  Operator=reciprocal  SaturateOnIntegerOverflow=on
  Multiport Switch : MultiPortSwitch  Inputs=2
  Product : Product  RndMeth=Zero
  Product1 : Product  RndMeth=Zero
  Saturation : Saturate  UpperLimit=inf  LowerLimit=0
  Sum : Sum  SaturateOnIntegerOverflow=on  InputSameDT=on  OutDataTypeStr=Inherit: Same as first input
  Sum1 : Sum  SaturateOnIntegerOverflow=on  InputSameDT=on  OutDataTypeStr=Inherit: Same as first input
  Trigonometric Function : Trigonometry  Operator=cos
  b0 : Gain  Gain=-b0  SaturateOnIntegerOverflow=on  OutDataTypeStr=Inherit: Same as input  ParamDataTypeStr=Inherit: Same as input
  b1 : Gain  Gain=-1/30  SaturateOnIntegerOverflow=on  OutDataTypeStr=Inherit: Same as input  ParamDataTypeStr=Inherit: Same as input
  qsolar : Outport
  Iglb : Outport  Port=2
  wires:
  Bias4/1 -> Product1/1
  Product1/1 -> Multiport Switch/3
  Constant/1 -> Product1/2
  b1/1 -> Bias4/1
  Bias3/1 -> b1/1
  Multiport Switch/1 -> Saturation/1
  Bias1/1 -> Multiport Switch/2
  Bias2/1 -> Multiport Switch/1
  Compare To Constant/1 -> Bias2/1
  Saturation/1 -> Product/1
  WDB/1 -> Bus Selector/1
  Bus Selector/3 -> IAM Kdiffuse/1, Sum1/2  "<Solar_Radiation_diffuse_surface>"
  Bus Selector/1 -> Degrees to Radians/1, Compare To Constant/1, Bias3/1  "<Incidence_Angle_sun>"
  Bus Selector/2 -> Product/2, Sum1/1  "<Solar_Radiation_direct_surface>"
  IAM Kdiffuse/1 -> Sum/2
  Product/1 -> Sum/1
  Sum/1 -> F'(tau*alfa)/1
  F'(tau*alfa)/1 -> qsolar/1
  Sum1/1 -> Iglb/1
  Degrees to Radians/1 -> Trigonometric Function/1
  Trigonometric Function/1 -> Math Function/1
  Math Function/1 -> Bias/1
  Bias/1 -> b0/1
  b0/1 -> Bias1/1

== system carnot/Source/Solar_Thermal/IncidenceAngleModifier/Theoretical_Collector_Optics ==
  WDB : Inport
  IAM_Table : $bdroot/Source/Solar_Thermal/IncidenceAngleModifier/IAM_Table  fta=FTA  angle=teta  Kb=kb  Kd=kd
  qsolar : Outport
  Iglb : Outport  Port=2
  wires:
  WDB/1 -> IAM_Table/1
  IAM_Table/1 -> qsolar/1
  IAM_Table/2 -> Iglb/1

== system carnot/Source/Solar_Thermal/PressureDropCollector/pressure_drop_calculated_data_water ==
  T : Inport
  mdot : Inport  Port=2
  p : Inport  Port=3
  lin_qua : Inport  Port=4
  1/acol : Gain  Gain=1/acol  SaturateOnIntegerOverflow=on  OutDataTypeStr=Inherit: Same as input  ParamDataTypeStr=Inherit: Same as input
  Aonecol : Gain  Gain=aonecol  SaturateOnIntegerOverflow=on  OutDataTypeStr=Inherit: Same as input  ParamDataTypeStr=Inherit: Same as input
  Demux3 : Demux  Outputs=2
  Look-Up Table (2-D) : Lookup2D  RowIndex=0:50:200  ColumnIndex=0:0.01:0.05  Table="[0 121.8750 261.8368 419.7212 595.443 788.9438; 0 44.3145 106.6853 186.9531 285.0355 400.8755; 0 29.8974 78.2964 145.0362 230.0334 333.2306; 0 24.2577 67.8077 130.4839 212.2001 312.8971; 0  21.7174 64.2104 127.3018 210.8995 314.9402]"  SaturateOnIntegerOverflow=on  InputSameDT=on
  Math Function : Math  Operator=square  SaturateOnIntegerOverflow=on
  Mux : Mux  Inputs=2
  Product : Product  Inputs=*/  SaturateOnIntegerOverflow=on  InputSameDT=on  OutDataTypeStr=Inherit: Same as first input
  Sum : Sum  Inputs=-+  SaturateOnIntegerOverflow=on  InputSameDT=on  OutDataTypeStr=Inherit: Same as first input
  Sum1 : Sum  SaturateOnIntegerOverflow=on  InputSameDT=on  OutDataTypeStr=Inherit: Same as first input
  p_out : Outport
  lq_out : Outport  Port=2
  wires:
  Look-Up Table (2-D)/1 -> Aonecol/1
  T/1 -> Look-Up Table (2-D)/1
  1/acol/1 -> Look-Up Table (2-D)/2
  mdot/1 -> 1/acol/1, Math Function/1
  lin_qua/1 -> Demux3/1
  Demux3/2 -> Sum1/2
  Sum1/1 -> Product/1
  Math Function/1 -> Product/2
  Product/1 -> Mux/2
  Mux/1 -> lq_out/1
  Demux3/1 -> Mux/1
  Sum/1 -> p_out/1
  p/1 -> Sum/2
  Aonecol/1 -> Sum/1, Sum1/1

== system carnot/Source/Solar_Thermal/PressureDropCollector/pressure_drop_for_measured_data_water ==
  T : Inport
  mdot : Inport  Port=2
  p : Inport  Port=3
  lin_qua : Inport  Port=4
  1/Ttest : Gain  Gain=1/ttest  SaturateOnIntegerOverflow=on  OutDataTypeStr=Inherit: Same as input  ParamDataTypeStr=Inherit: Same as input
  Aonecol/ (Acol*mdottest) : Gain  Gain=aonecol/(acol*mdottest)  SaturateOnIntegerOverflow=on  OutDataTypeStr=Inherit: Same as input  ParamDataTypeStr=Inherit: Same as input
  Demux3 : Demux  Outputs=2
  Look-Up Table (2-D) : Lookup2D  RowIndex=0:2.5:10  ColumnIndex=0:0.6175:3.0875  Table="pdroptest*[0  0.7699  1.6541  2.6516  3.7617  4.9841;  0  0.28  0.674  1.1811  1.8007  2.5325;  0  0.1889  0.4946  0.9163  1.4532  2.1052;  0  0.1532  0.4284  0.8243  1.3406  1.9767;  0  0.1372  0.4056  0.8042  1.3323  1.9896]"  SaturateOnIntegerOverflow=on  InputSameDT=on
  Math Function : Math  Operator=square  SaturateOnIntegerOverflow=on
  Mux : Mux  Inputs=2
  Product : Product  Inputs=*/  SaturateOnIntegerOverflow=on  InputSameDT=on  OutDataTypeStr=Inherit: Same as first input
  Sum : Sum  Inputs=-+  SaturateOnIntegerOverflow=on  InputSameDT=on  OutDataTypeStr=Inherit: Same as first input
  Sum1 : Sum  SaturateOnIntegerOverflow=on  InputSameDT=on  OutDataTypeStr=Inherit: Same as first input
  p_out : Outport
  lq_out : Outport  Port=2
  wires:
  Aonecol/ (Acol*mdottest)/1 -> Look-Up Table (2-D)/2
  1/Ttest/1 -> Look-Up Table (2-D)/1
  T/1 -> 1/Ttest/1
  lin_qua/1 -> Demux3/1
  Demux3/2 -> Sum1/2
  Sum1/1 -> Product/1
  Math Function/1 -> Product/2
  Product/1 -> Mux/2
  Mux/1 -> lq_out/1
  Demux3/1 -> Mux/1
  Sum/1 -> p_out/1
  p/1 -> Sum/2
  Look-Up Table (2-D)/1 -> Sum/1, Sum1/1
  mdot/1 -> Aonecol/ (Acol*mdottest)/1, Math Function/1

== system carnot/Source/Solar_Thermal/PressureDropCollector/pressure_drop_quadratic_fitted_data ==
  T : Inport
  mdot : Inport  Port=2
  p : Inport  Port=3
  lin_qua : Inport  Port=4
  Aonecol/Acol : Gain  Gain=aonecol/acol  SaturateOnIntegerOverflow=on  OutDataTypeStr=Inherit: Same as input  ParamDataTypeStr=Inherit: Same as input
  Demux3 : Demux  Outputs=2
  Mux : Mux  Inputs=2
  Sum : Sum  Inputs=-+  SaturateOnIntegerOverflow=on  InputSameDT=on  OutDataTypeStr=Inherit: Same as first input
  Sum1 : Sum  SaturateOnIntegerOverflow=on  InputSameDT=on  OutDataTypeStr=Inherit: Same as first input
  Sum2 : Sum  SaturateOnIntegerOverflow=on  InputSameDT=on  OutDataTypeStr=Inherit: Same as first input
  T-correction : Lookup  InputValues=[0 400]  Table=[1 1]  SaturateOnIntegerOverflow=on
  const : Constant  Value=b
  const1 : Constant  Value=a
  dp per collector : DotProduct  OutDataTypeStr=Inherit: Inherit via internal rule
  pressuredrop : Fcn  Expr=(a*u[1]+b)*u[1]
  p_out : Outport
  lq_out : Outport  Port=2
  wires:
  mdot/1 -> Aonecol/Acol/1
  Aonecol/Acol/1 -> pressuredrop/1
  T/1 -> T-correction/1
  Sum2/1 -> Mux/1
  const1/1 -> Sum1/1
  const/1 -> Sum2/1
  Demux3/1 -> Sum2/2
  Sum1/1 -> Mux/2
  Sum/1 -> p_out/1
  dp per collector/1 -> Sum/1
  p/1 -> Sum/2
  Mux/1 -> lq_out/1
  Demux3/2 -> Sum1/2
  lin_qua/1 -> Demux3/1
  T-correction/1 -> dp per collector/1
  pressuredrop/1 -> dp per collector/2

== system carnot/Source/Solar_Thermal/PressureDropCollector/pressure_drop_quadratic_fitted_data_water ==
  T : Inport
  mdot : Inport  Port=2
  p : Inport  Port=3
  lin_qua : Inport  Port=4
  Aonecol/Acol : Gain  Gain=aonecol/acol  SaturateOnIntegerOverflow=on  OutDataTypeStr=Inherit: Same as input  ParamDataTypeStr=Inherit: Same as input
  Demux3 : Demux  Outputs=2
  Mux : Mux  Inputs=2
  Sum : Sum  Inputs=-+  SaturateOnIntegerOverflow=on  InputSameDT=on  OutDataTypeStr=Inherit: Same as first input
  Sum1 : Sum  SaturateOnIntegerOverflow=on  InputSameDT=on  OutDataTypeStr=Inherit: Same as first input
  Sum2 : Sum  SaturateOnIntegerOverflow=on  InputSameDT=on  OutDataTypeStr=Inherit: Same as first input
  T-correction fluid Water : Lookup  InputValues=0:20:200  Table="[0.9985  1.0  1.006  1.0154  1.0275  1.0419  1.0590  1.0794  1.1045  1.1367  1.1795]"  SaturateOnIntegerOverflow=on
  const : Constant  Value=b
  const1 : Constant  Value=a
  dp per collector : DotProduct  InputSameDT=on  OutDataTypeStr=Inherit: Inherit via internal rule
  pressuredrop : Fcn  Expr=(a*u[1]+b)*u[1]
  p_out : Outport
  lq_out : Outport  Port=2
  wires:
  pressuredrop/1 -> dp per collector/2
  T-correction fluid Water/1 -> dp per collector/1
  lin_qua/1 -> Demux3/1
  Demux3/2 -> Sum1/2
  Mux/1 -> lq_out/1
  p/1 -> Sum/2
  dp per collector/1 -> Sum/1
  Sum/1 -> p_out/1
  Sum1/1 -> Mux/2
  Demux3/1 -> Sum2/2
  const/1 -> Sum2/1
  const1/1 -> Sum1/1
  Sum2/1 -> Mux/1
  T/1 -> T-correction fluid Water/1
  Aonecol/Acol/1 -> pressuredrop/1
  mdot/1 -> Aonecol/Acol/1

== system carnot/Source/Solar_Thermal/SolarCollector/create_Cdat ==
  acol : Inport
  THBin : Inport  Port=2
  THBout : Inport  Port=3
  Qdot : Inport  Port=4
  Tmean : Inport  Port=5
  WDB : Inport  Port=6
  Bus Creator : BusCreator  Inputs=6
  Cdat : Outport
  wires:
  acol/1 -> Bus Creator/1  "Acol"
  THBin/1 -> Bus Creator/2  "THBin"
  THBout/1 -> Bus Creator/3  "THBout"
  WDB/1 -> Bus Creator/6  "WDB_surface"
  Bus Creator/1 -> Cdat/1
  Qdot/1 -> Bus Creator/4  "Qdot"
  Tmean/1 -> Bus Creator/5  "Tmean"
